simulink model "mathmodel"  (R2022b)
settings: Solver=VariableStepAuto  StartTime=0.0  StopTime=1.0  RelTol=1e-3
values from neighbouring files (symbols this model uses):
  J = (15.6 / 1000) * (22.49 / 1000 / 2)^2 / 2 * 48^2    (= 0.00227245868928)    [UI.m]
  Ke = (ke_p + ke_n) / 2    [UI.m]
  Km = Ke    [UI.m]
  L = 0.0047    [UI.m]
  R = (R_n + R_p) / 2    [UI.m]
  U_pr = Uall(i)    [UI.m]
settings Model: Creator=tameembourgi  LastModifiedBy=Alena

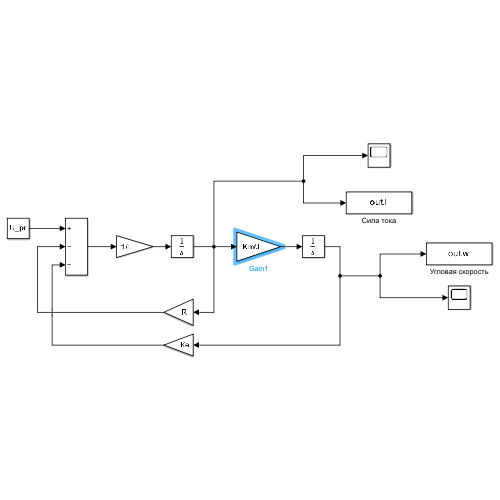
[thumbnail: Simulink's stored preview of the top-level diagram]
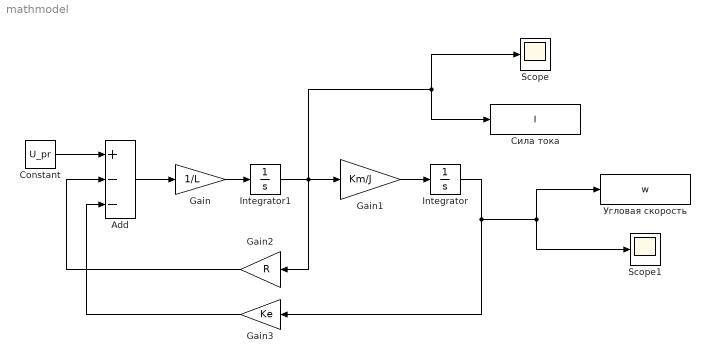
== system mathmodel ==
  Add : Sum  Inputs=+--
  Constant : Constant  Value=U_pr
  Gain : Gain  Gain=1/L
  Gain1 : Gain  Gain=Km/J
  Gain2 : Gain  Gain=R
  Gain3 : Gain  Gain=Ke
  Integrator : Integrator
  Integrator1 : Integrator
  Scope : Scope
  Scope1 : Scope
  Сила тока : ToWorkspace  VariableName=I  SaveFormat=Timeseries  SampleTime=-1
  Угловая скорость : ToWorkspace  VariableName=w  SaveFormat=Timeseries  SampleTime=-1
  wires:
  Constant/1 -> Add/1
  Add/1 -> Gain/1
  Gain/1 -> Integrator1/1
  Integrator1/1 -> Сила тока/1, Scope/1, Gain2/1, Gain1/1
  Gain1/1 -> Integrator/1
  Integrator/1 -> Gain3/1, Scope1/1, Угловая скорость/1
  Gain3/1 -> Add/3
  Gain2/1 -> Add/2
